simulink model "A04_L9_2"  (R2014b)
settings: Solver=ode45  StartTime=0.0  StopTime=10.0  RelTol=1e-3
settings Model: Creator=User  LastModifiedBy=User

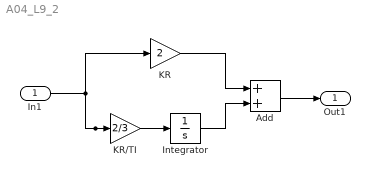
== system A04_L9_2 ==
  In1 : Inport
  Add : Sum
  Integrator : Integrator
  KR : Gain  Gain=2
  KR/TI : Gain  Gain=2/3
  Out1 : Outport
  wires:
  Add/1 -> Out1/1
  KR/1 -> Add/1
  Integrator/1 -> Add/2
  In1/1 -> KR/TI/1, KR/1
  KR/TI/1 -> Integrator/1
